simulink model "Enslavement"  (R2014a)
settings: Solver=ode45  StartTime=0.0  StopTime=0.01  RelTol=1e-3
settings Model: Creator=Farad  LastModifiedBy=Farad

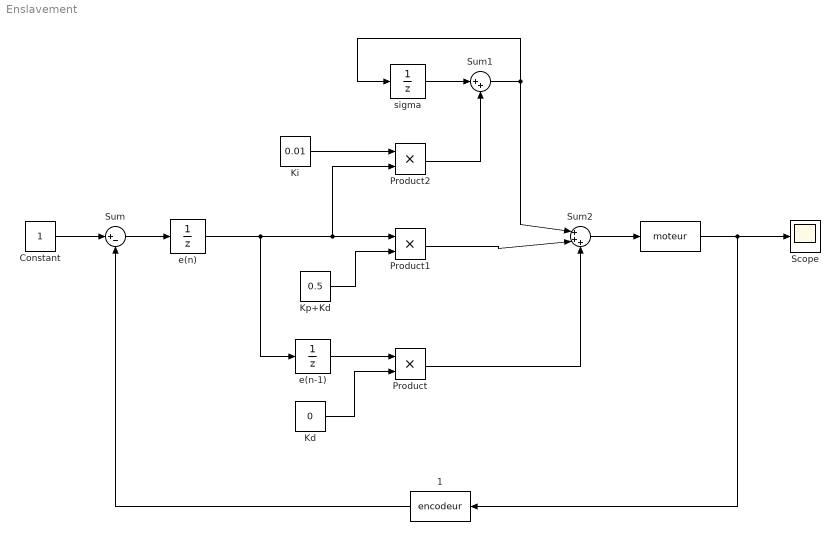
== system Enslavement ==
  " " : Fcn  Expr=moteur
  " 1" : Fcn  Expr=encodeur
  Constant : Constant
  Kd : Constant  Value=0
  Ki : Constant  Value=0.01
  Kp+Kd : Constant  Value=0.5
  Product : Product
  Product1 : Product
  Product2 : Product
  Scope : Scope
  Sum : Sum  Inputs=|+-
  Sum1 : Sum  Inputs=|++
  Sum2 : Sum  Inputs=|+++
  e(n) : UnitDelay  SampleTime=-1
  "e(n-1) " : UnitDelay  SampleTime=-1
  "sigma " : UnitDelay  SampleTime=-1
  wires:
  Constant/1 -> Sum/1
  Sum/1 -> e(n)/1
  "e(n-1) "/1 -> Product/1
  Kd/1 -> Product/2
  Kp+Kd/1 -> Product1/2
  Product2/1 -> Sum1/2
  "sigma "/1 -> Sum1/1
  Product1/1 -> Sum2/2
  Product/1 -> Sum2/3
  Ki/1 -> Product2/1
  e(n)/1 -> Product1/1, Product2/2, "e(n-1) "/1
  Sum1/1 -> "sigma "/1, Sum2/1
  Sum2/1 -> " "/1
  " "/1 -> " 1"/1, Scope/1
  " 1"/1 -> Sum/2
